simulink model "c_coder"  (R2021b)
settings: Solver=FixedStepAuto  StartTime=0.0  StopTime=inf  FixedStep=0.02  RelTol=1e-3
InitFcn:
  | run('./init_simulink.m');
values from neighbouring files (symbols this model uses):
  qsi = 1    [init_simulink.m]
  w0_acc = 2*pi*f0_acc    (= 0.628318530718)    [init_simulink.m]
  w0_lp = 2*pi*f0_lp    (= 6.28318530718)    [init_simulink.m]
  w0_pos = 2*pi*f0_pos    (= 6.28318530718)    [init_simulink.m]
  w0_vel = 2*pi*f0_vel    (= 1.88495559215)    [init_simulink.m]
undefined symbols (not defined in the file or in its folder): CR, DiscIntNeverNeededParam, LF
libraries: dspstat3 x6, simulink x3, slrealtimeiplib x3, instrumentlib x2, instrumentseriallib x2, etargetslib x1, simulink_extras x1, aerolibanimutils x1, dspnetwork x1
settings Model: Creator=sergi  LastModifiedBy=filip
settings SolverCC: AllowMultiTaskInputOutput=on  AlgebraicLoopSolver=TrustRegion  PositivePriorityOrder=on  AutoInsertRateTranBlk=on
settings DataIOCC: ReturnWorkspaceOutputs=off
settings OptimizationCC: BlockReduction=off  DefaultParameterBehavior=Inlined  EnhancedBackFolding=on  PassReuseOutputArgsAs=Individual arguments  ZeroExternalMemoryAtStartup=off  OptimizeBlockOrder=speed  DifferentSizesBufferReuse=on  OptimizationCustomize=off  EfficientTunableParamExpr=on
settings DebuggingCC: TasksWithSamePriorityMsg=none  ParameterTunabilityLossMsg=error  SFMachineParentedDataDiag=warning  ArithmeticOperatorsInVariantConditions=warning
settings HardwareCC: TargetBitPerPointer=64  TargetBitPerSizeT=64  TargetBitPerPtrDiffT=64  TargetLongLongMode=on  TargetIntDivRoundTo=Zero  TargetEndianess=LittleEndian  TargetWordSize=64  TargetHWDeviceType=MATLAB Host  ProdEqTarget=off
settings SFSimCC: SimUseLocalCustomCode=off  MATLABDynamicMemAlloc=off  CustomCodeUndefinedFunction=UseInterfaceOnly
settings RTWCC: Description=Embedded Coder (host-based shared library target)  SystemTargetFile=ert_shrlib.tlc  TemplateMakefile=ert_default_tmf  GenerateReport=on  RTWUseLocalCustomCode=off  Toolchain=MinGW64 | gmake (64-bit Windows)  BuildConfiguration=Faster Runs  LaunchReport=on  CodeExecutionProfiling=on
settings CodeAppCC: ForceParamTrailComments=on  IgnoreCustomStorageClasses=off  MaxIdLength=95  OperatorAnnotations=on  SimulinkDataObjDesc=on  SFDataObjDesc=on  InsertBlockDesc=on
settings STFCustomTargetCC: TargetLangStandard=C99 (ISO)  MultiwordLength=256  GenerateSampleERTMain=on  ParMdlRefBuildCompliant=on  CompOptLevelCompliant=on  CombineOutputUpdateFcns=on  ERTCustomFileBanners=on  CodeInterfacePackaging=Reusable function  SupportNonInlinedSFcns=off  RemoveResetFunc=on  MATLABClassNameForMDSCustomization=Simulink.SoftwareTarget.ERTCustomization  ModelStepFunctionPrototypeControlCompliant=on  GRTInterface=off  UseToolchainInfoCompliant=on  SystemTargetFile=ert_shrlib.tlc
settings ERTTargetCC: TargetLangStandard=C99 (ISO)  GenerateSampleERTMain=on  ConcurrentExecutionCompliant=off  CodeInterfacePackaging=Reusable function  SupportContinuousTime=on  CPPClassGenCompliant=off  InlinedParameterPlacement=NonHierarchical  ERTCustomFileTemplate=example_file_process.tlc

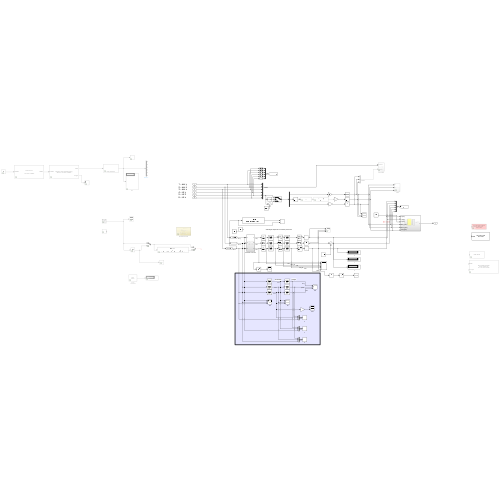
[thumbnail: Simulink's stored preview of the top-level diagram]
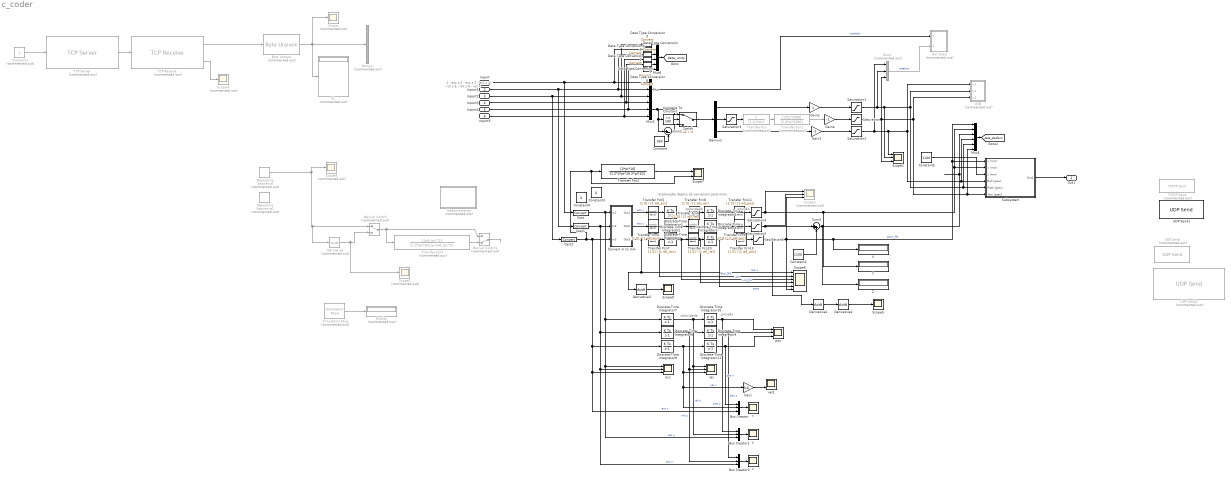
== system c_coder ==
  note: 1 - acc y
      | 2 - acc z
      | 3 - acc x
      | 4 - rot y
      | 5 - rot z
      | 6 - rot x
  note: aceleração depois da conversao para mms
  note: posição
  note: velocidade
  note: posição
  note: velocidade
  Inport : Inport  OutDataTypeStr=double
  Inport1 : Inport  Port=2  OutDataTypeStr=double
  Inport2 : Inport  Port=3  OutDataTypeStr=double
  Inport3 : Inport  Port=4  OutDataTypeStr=double
  Inport4 : Inport  Port=5  OutDataTypeStr=double
  Inport5 : Inport  Port=6  OutDataTypeStr=double
  Bus Creator : BusCreator  Inputs=3
  Bus Creator1 : BusCreator  Inputs=3
  Bus Creator2 : BusCreator  Inputs=3
  Byte Unpack : etargetslib/Byte Unpack  Commented=on  dimensions={[6]}  datatypes={'single'}  byteAlign=1
  Cast : DataTypeConversion
  Cast1 : DataTypeConversion
  Cast2 : DataTypeConversion
  Compare To Constant : simulink/Logic and Bit Operations/Compare To Constant  relop=<=  const=180  OutDataTypeStr=boolean
  Constant : Constant  Value=360
  Constant1 : Constant  Commented=on
  Constant2 : Constant  Value=1100
  Constant3 : Constant  Value=0
  Constant4 : Constant  Value=0
  Constant5 : Constant  Value=1100
  Convert m to mm : Subsystem
  Data Type Conversion{3..8} (6 alike) : DataTypeConversion
  Demux : Demux  Commented=on  Outputs=6
  Demux1 : Demux  Outputs=3
  Derivative : Derivative  Commented=on
  Derivative1 : Derivative
  Derivative2 : Derivative
  Derivative3 : Derivative
  Discrete-Time Integrator{,2..11} (11 alike) : DiscreteIntegrator  SampleTime=-1  UpperSaturationLimit=150  LowerSaturationLimit=-150  ICPrevOutput=DiscIntNeverNeededParam  ICPrevScaledInput=DiscIntNeverNeededParam
  Discrete-Time Integrator1 : DiscreteIntegrator  SampleTime=-1  UpperSaturationLimit=1000  LowerSaturationLimit=-1000  ICPrevOutput=DiscIntNeverNeededParam  ICPrevScaledInput=DiscIntNeverNeededParam
  Display : Display  Commented=on
  Gain : Gain  Gain=3.6
  Gain2 : Gain
  Gain3 : Gain  Gain=-1
  Gain4 : Gain  Gain=-1
  Manual Switch : ManualSwitch  Commented=on
  Manual Switch1 : ManualSwitch  Commented=on  CurrentSetting=0
  Measurements : Subsystem  Commented=on
  Mux : Mux  Inputs=3
  Mux1 : Mux  Commented=on  Inputs=3
  Mux2 : Mux  Inputs=3
  Mux5 : Mux  Inputs=6
  Mux6 : Mux  Inputs=6
  Not Used : Subsystem  Commented=on
  Repeating Sequence : simulink/Sources/Repeating Sequence  Commented=on  rep_seq_t=[0 2 10 17 21 23 30 39 45 50]  rep_seq_y=[0 0 2.4 2.4 -0.33 -0.33 -5.8 -5.8 0 0]
  Repeating Sequence1 : simulink/Sources/Repeating Sequence  Commented=on  rep_seq_t=t_acc  rep_seq_y=v_acc
  Saturation{,1..3} (4 alike) : Saturate  UpperLimit=15  LowerLimit=-15
  Saturation4 : Saturate  UpperLimit=250  LowerLimit=-250
  Saturation5 : Saturate  UpperLimit=250  LowerLimit=-250
  Saturation6 : Saturate  UpperLimit=250  LowerLimit=-250
  Scope{,2,4,8} (4 alike) : Scope  Commented=on
  Scope1 : Scope  NumInputPorts=3
  Scope3 : Scope  Commented=on  NumInputPorts=3
  Scope5 : Scope
  Scope6 : Scope  NumInputPorts=6
  Scope7 : Scope  NumInputPorts=2
  Scope9 : Scope
  Simulation Pace : aerolibanimutils/Simulation Pace  Commented=on  SimulationPace=1  SleepMode=Auto  OutputPaceError=on  SampleTime=0.02
  Subsystem : Subsystem
  Sum2 : Sum  Inputs=|+-
  Sum3 : Sum  Inputs=|++
  Switch : Switch  Criteria=u2 > Threshold
  TCP Receive : slrealtimeiplib/TCP Receive  Commented=on  socketAddPortVal=<empty>  rcvWidth=6*4  sampleTime=-1
      settings: SourceProductBaseCode=XP
  TCP Server : slrealtimeiplib/TCP Server  Priority=-1  Commented=on  useHostTargetConn=off  serverAddress=127.0.0.1  serverPort=55001
      settings: SourceProductBaseCode=XP
  TCP/IP Send : instrumentlib/TCP//IP Send  Commented=on  Host=192.168.0.101  Port=502  ByteOrder=little-endian  EnableBlockingMode=off  Timeout=10  TransferDelay=on  SimulateUsing=Interpreted execution
  Transfer Fcn : TransferFcn  Commented=on  Numerator=[1 0]  Denominator=[1 0.2*pi]
  Transfer Fcn1 : TransferFcn  Commented=on  Numerator=[2*pi*1000]  Denominator=[1 2*pi*1000]
  Transfer Fcn10 : TransferFcn  Numerator=[1 0]  Denominator=[1 w0_vel]
  Transfer Fcn11 : TransferFcn  Numerator=[1 0]  Denominator=[1 w0_pos]
  Transfer Fcn13 : TransferFcn  Numerator=[1 0]  Denominator=[1 w0_pos]
  Transfer Fcn2 : TransferFcn  Numerator=[2*pi*10]  Denominator=[1 2*2*pi*10 2*pi*10]
  Transfer Fcn3 : TransferFcn  Commented=on  Numerator=[(w0_lp)^2]  Denominator=[1 2*qsi*w0_lp (w0_lp)^2]
  Transfer Fcn4 : TransferFcn  Numerator=[1 0]  Denominator=[1 w0_acc]
  Transfer Fcn5 : TransferFcn  Numerator=[1 0]  Denominator=[1 w0_acc]
  Transfer Fcn6 : TransferFcn  Numerator=[1 0]  Denominator=[1 w0_vel]
  Transfer Fcn7 : TransferFcn  Numerator=[1 0]  Denominator=[1 w0_acc]
  Transfer Fcn8 : TransferFcn  Numerator=[1 0]  Denominator=[1 w0_vel]
  Transfer Fcn9 : TransferFcn  Numerator=[1 0]  Denominator=[1 w0_pos]
  UDP Send : dspnetwork/UDP Send  Commented=on  remoteURL='127.0.0.1'  remotePort=25000  localURL='0.0.0.0'  localPortSource=Automatically determine  localPort=-1  sendBufferSize=8192  sampletime=-1  blockPlatform=[]  separateLengthPort=0
  UDP Send1 : instrumentlib/UDP Send  Host=192.168.0.100  Port=502  LocalPort=-1  EnablePortSharing=off  ByteOrder=LittleEndian  OutputDatagramPacketSize=256  EnableBlockingMode=on  LocalAddress=0.0.0.0
  UDP Send2 : slrealtimeiplib/UDP Send  Commented=on  useHostTargetConn=off  toAddress='10.10.10.10'  toPort=34  sampleTime=-1
      settings: SourceProductBaseCode=XP
  USB : Subsystem  Commented=on
  X : Display
  X1 : Display  Commented=on
  Y : Display
  Z : Display
  acc : Scope  NumInputPorts=3
  pos : Scope  NumInputPorts=3
  vel : Scope  NumInputPorts=3
  vel1 : Scope  NumInputPorts=3
  x : Scope
  y : Scope
  z : Scope
  Out1 : Outport
  tag scope: data_platform=global, data_unity=global
  wires:
  Inport5/1 -> Mux2/3, Data Type Conversion6/1
  Inport3/1 -> Data Type Conversion7/1, Mux2/1
  Inport2/1 -> Cast2/1, Mux/3, Data Type Conversion3/1
  Inport1/1 -> Cast1/1, Data Type Conversion5/1, Mux/2
  Inport/1 -> Data Type Conversion4/1, Mux/1, Cast/1
  Mux2/1 -> Switch/1, Sum2/1, Compare To Constant/1
  Constant/1 -> Sum2/2
  Compare To Constant/1 -> Switch/2
  Sum2/1 -> Switch/3
  Demux1/1 -> Gain2/1
  Demux1/3 -> Gain3/1
  Transfer Fcn/1 -> Transfer Fcn1/1
  Demux1/2 -> Saturation3/1
  Saturation1/1 -> Scope1/2, Subsystem/5(Pitch (grau)), Mux5/5, USB/2(In2), Mux1/2
  Saturation2/1 -> Mux1/1, USB/1(In1), Subsystem/4("Roll (grau) "), Mux5/4, Scope1/1
  Gain2/1 -> Saturation1/1
  Gain3/1 -> Saturation2/1
  Saturation3/1 -> Transfer Fcn/1
  Switch/1 -> Demux1/1
  Saturation/1 -> Scope1/3, Subsystem/6(Yaw (grau)), Mux5/6, USB/3(In3), Mux1/3
  Transfer Fcn1/1 -> Gain4/1
  Gain4/1 -> Saturation/1
  Mux5/1 -> [data_platform]
  Inport4/1 -> Data Type Conversion8/1, Mux2/2
  Data Type Conversion3/1 -> Mux6/1
  Data Type Conversion4/1 -> Mux6/2
  Data Type Conversion5/1 -> Mux6/3
  Data Type Conversion6/1 -> Mux6/4
  Data Type Conversion7/1 -> Mux6/5
  Data Type Conversion8/1 -> Mux6/6
  Mux6/1 -> [data_unity]
  Mux/1 -> Not Used/1(position)  "position"
  Mux1/1 -> Not Used/2(rotation)  "rotation"
  Subsystem/1(Out1) -> Out1/1
  Discrete-Time Integrator1/1 -> Transfer Fcn8/1
  Discrete-Time Integrator/1 -> Transfer Fcn6/1
  Discrete-Time Integrator2/1 -> Scope6/3, Transfer Fcn10/1  "velx"
  Discrete-Time Integrator4/1 -> Transfer Fcn11/1
  Discrete-Time Integrator3/1 -> Transfer Fcn9/1
  Discrete-Time Integrator5/1 -> Scope6/5, Transfer Fcn13/1  "posx"
  Cast/1 -> acc/1, Bus Creator1/3, Discrete-Time Integrator7/1, Convert m to mm/1(In1)  "acc y"
  Cast1/1 -> Convert m to mm/2(In2), Bus Creator2/3, acc/2, Discrete-Time Integrator6/1  "acc z"
  Cast2/1 -> Scope7/2, Transfer Fcn2/1, Discrete-Time Integrator8/1, Bus Creator/3, acc/3, Convert m to mm/3(In3)  "acc x"
  Saturation4/1 -> Scope3/1, Y/1, Subsystem/2(y (mm)), Mux5/2
  Sum3/1 -> Mux5/3, Z/1
  Saturation6/1 -> Derivative1/1, Scope3/3, Scope6/6, X/1, Subsystem/1(x (mm)), Mux5/1  "posx_filt"
  Constant2/1 -> Sum3/2
  Saturation5/1 -> Scope3/2, Sum3/1
  Convert m to mm/1(Out1) -> Transfer Fcn5/1  "acc y"
  Convert m to mm/2(Out2) -> Transfer Fcn4/1  "acc z"
  Convert m to mm/3(Out3) -> Scope6/1, Derivative3/1, Transfer Fcn7/1  "acc x"
  TCP Receive/2 -> Scope4/1
  Constant1/1 -> TCP Server/1
  TCP Server/1 -> TCP Receive/1
  Byte Unpack/1 -> Demux/1, Scope/1, X1/1
  Discrete-Time Integrator11/1 -> Bus Creator/1, pos/3  "pos x"
  Discrete-Time Integrator9/1 -> Bus Creator2/1, pos/2  "pos z"
  Discrete-Time Integrator10/1 -> Bus Creator1/1, pos/1  "pos y"
  Discrete-Time Integrator8/1 -> Discrete-Time Integrator11/1, Bus Creator/2, Gain/1, vel/3  "vel x"
  Discrete-Time Integrator6/1 -> Discrete-Time Integrator9/1, Bus Creator2/2, vel/2  "vel z"
  Discrete-Time Integrator7/1 -> Discrete-Time Integrator10/1, Bus Creator1/2, vel/1  "vel y"
  Bus Creator/1 -> x/1
  Bus Creator1/1 -> y/1
  Bus Creator2/1 -> z/1
  Transfer Fcn5/1 -> Discrete-Time Integrator1/1
  Transfer Fcn4/1 -> Discrete-Time Integrator/1
  Transfer Fcn7/1 -> Scope6/2, Discrete-Time Integrator2/1  "accx_filt"
  Transfer Fcn6/1 -> Discrete-Time Integrator3/1
  Transfer Fcn10/1 -> Scope6/4, Discrete-Time Integrator5/1  "vrlx_filt"
  Transfer Fcn8/1 -> Discrete-Time Integrator4/1
  Transfer Fcn13/1 -> Saturation6/1
  Transfer Fcn9/1 -> Saturation5/1
  Transfer Fcn11/1 -> Saturation4/1
  Constant5/1 -> Subsystem/3(z (mm))
  Transfer Fcn2/1 -> Scope7/1
  Repeating Sequence/1 -> Scope8/1, Derivative/1, Manual Switch/1
  Manual Switch/1 -> Manual Switch1/1, Transfer Fcn3/1
  Derivative/1 -> Scope2/1, Manual Switch/2
  Manual Switch1/1 -> ?
  Transfer Fcn3/1 -> Manual Switch1/2
  Derivative1/1 -> Derivative2/1
  Derivative2/1 -> Scope5/1
  Derivative3/1 -> Scope9/1
  Simulation Pace/1 -> Display/1
  Gain/1 -> vel1/3
  TCP Receive/1 -> Byte Unpack/1

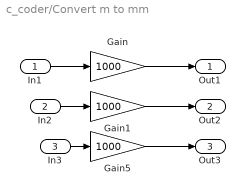
== system c_coder/Convert m to mm ==
  In1 : Inport
  In2 : Inport  Port=2
  In3 : Inport  Port=3
  Gain : Gain  Gain=1000
  Gain1 : Gain  Gain=1000
  Gain5 : Gain  Gain=1000
  Out1 : Outport
  Out2 : Outport  Port=2
  Out3 : Outport  Port=3
  wires:
  Gain/1 -> Out1/1
  Gain5/1 -> Out3/1
  In3/1 -> Gain5/1
  In1/1 -> Gain/1
  In2/1 -> Gain1/1
  Gain1/1 -> Out2/1

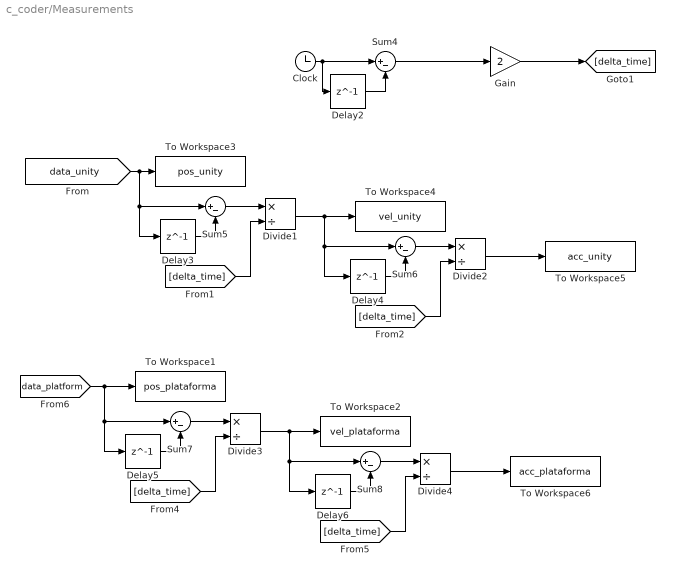
== system c_coder/Measurements ==
  Clock : Clock
  Delay{2..6} (5 alike) : Delay  DelayLength=1
  Divide{1..4} (4 alike) : Product  Inputs=*/
  Gain : Gain  Gain=2
  Sum{4..8} (5 alike) : Sum  Inputs=|+-
  To Workspace1 : ToWorkspace  VariableName=pos_plataforma  SaveFormat=Structure With Time  SampleTime=-1
  To Workspace2 : ToWorkspace  VariableName=vel_plataforma  SaveFormat=Structure With Time  SampleTime=-1
  To Workspace3 : ToWorkspace  VariableName=pos_unity  SaveFormat=Structure With Time  SampleTime=-1
  To Workspace4 : ToWorkspace  VariableName=vel_unity  SaveFormat=Structure With Time  SampleTime=-1
  To Workspace5 : ToWorkspace  VariableName=acc_unity  SaveFormat=Structure With Time  SampleTime=-1
  To Workspace6 : ToWorkspace  VariableName=acc_plataforma  SaveFormat=Structure With Time  SampleTime=-1
  wires:
  Divide3/1 -> To Workspace2/1, Delay6/1, Sum8/1
  Divide2/1 -> To Workspace5/1
  Sum5/1 -> Divide1/1
  [delta_time] -> Divide1/2
  [data_unity] -> Delay3/1, Sum5/1, To Workspace3/1
  Delay2/1 -> Sum4/2
  Clock/1 -> Delay2/1, Sum4/1
  Delay3/1 -> Sum5/2
  [delta_time] -> Divide3/2
  [data_platform] -> To Workspace1/1, Sum7/1, Delay5/1
  Delay4/1 -> Sum6/2
  Divide1/1 -> Sum6/1, Delay4/1, To Workspace4/1
  Sum6/1 -> Divide2/1
  Sum7/1 -> Divide3/1
  [delta_time] -> Divide2/2
  Sum4/1 -> Gain/1
  [delta_time] -> Divide4/2
  Delay6/1 -> Sum8/2
  Divide4/1 -> To Workspace6/1
  Sum8/1 -> Divide4/1
  Delay5/1 -> Sum7/2
  Gain/1 -> [delta_time]

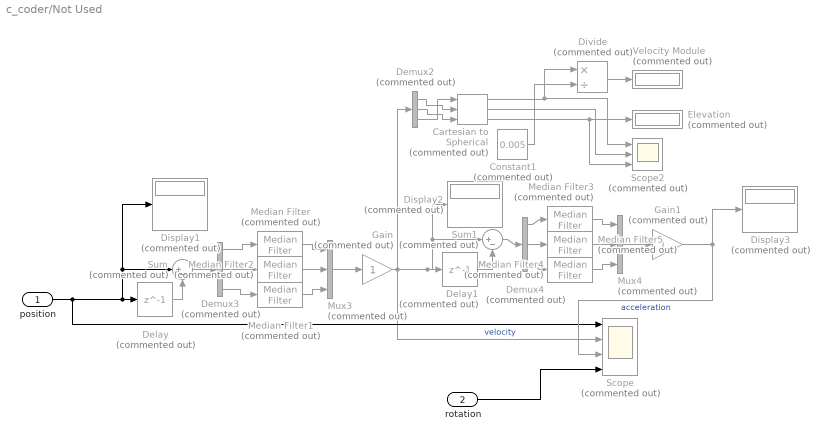
== system c_coder/Not Used ==
  position : Inport
  rotation : Inport  Port=2
  Cartesian to Spherical : simulink_extras/Transformations/Cartesian to Spherical  Commented=on
      settings: SourceProductBaseCode=SL
  Constant1 : Constant  Commented=on  Value=0.005
  Delay : Delay  Commented=on  DelayLength=1
  Delay1 : Delay  Commented=on  DelayLength=1
  Demux2 : Demux  Commented=on  Outputs=3
  Demux3 : Demux  Commented=on  Outputs=3
  Demux4 : Demux  Commented=on  Outputs=3
  Display1 : Display  Commented=on
  Display2 : Display  Commented=on
  Display3 : Display  Commented=on
  Divide : Product  Commented=on  Inputs=*/
  Elevation : Display  Commented=on
  Gain : Gain  Commented=on
  Gain1 : Gain  Commented=on
  Median Filter{,1..5} (6 alike) : dspstat3/Median Filter  Commented=on  WindowLength=10  SimulateUsing=Interpreted execution
      settings: SourceProductName=DSP System Toolbox
  Mux3 : Mux  Commented=on  Inputs=3
  Mux4 : Mux  Commented=on  Inputs=3
  Scope : Scope  Commented=on  NumInputPorts=4
  Scope2 : Scope  Commented=on  NumInputPorts=3
  Sum : Sum  Commented=on  Inputs=|+-
  Sum1 : Sum  Commented=on  Inputs=|+-
  Velocity Module : Display  Commented=on
  wires:
  Gain/1 -> Demux2/1, Scope/2, Display2/1, Sum1/1, Delay1/1  "velocity"
  Cartesian to Spherical/3 -> Scope2/3, Elevation/1
  position/1 -> Scope/1, Delay/1, Display1/1, Sum/1
  Delay/1 -> Sum/2
  Demux2/2 -> Cartesian to Spherical/3
  Demux3/3 -> Median Filter1/1
  Median Filter1/1 -> Mux3/3
  Median Filter4/1 -> Mux4/3
  Cartesian to Spherical/1 -> Scope2/1, Divide/1
  Gain1/1 -> Display3/1, Scope/3  "acceleration"
  Delay1/1 -> Sum1/2
  Demux3/2 -> Median Filter2/1
  Demux2/1 -> Cartesian to Spherical/2
  Demux3/1 -> Median Filter/1
  Sum/1 -> Demux3/1
  Median Filter5/1 -> Mux4/2
  Demux4/3 -> Median Filter4/1
  Mux3/1 -> Gain/1
  Mux4/1 -> Gain1/1
  Constant1/1 -> Divide/2
  Median Filter2/1 -> Mux3/2
  Demux2/3 -> Cartesian to Spherical/1
  Demux4/2 -> Median Filter5/1
  Sum1/1 -> Demux4/1
  Median Filter3/1 -> Mux4/1
  Median Filter/1 -> Mux3/1
  Demux4/1 -> Median Filter3/1
  Divide/1 -> Velocity Module/1
  Cartesian to Spherical/2 -> Scope2/2
  rotation/1 -> Scope/4

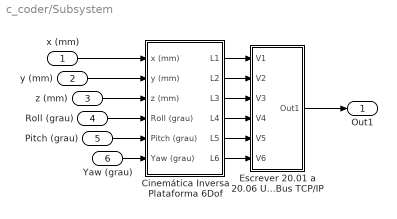
== system c_coder/Subsystem ==
  x (mm) : Inport
  y (mm) : Inport  Port=2
  z (mm) : Inport  Port=3
  "Roll (grau) " : Inport  Port=4
  Pitch (grau) : Inport  Port=5
  Yaw (grau) : Inport  Port=6
  Cinemática Inversa Plataforma 6Dof : Subsystem  mask(Cinemática Inversa - Plataforma 6DOF){a=180, b=180, c=1200, d=210, e=220, f=690, Lmin=750, Gs=10}
      mask prompts: a "Constante 'a' (mm)"; b "Constante 'b' (mm)"; c "Constante 'c' (mm)"; d "Constante 'd' (mm)"; e "Constante 'e (mm)"; f "Constante 'f' (mm)"; Lmin "Constante 'Lmin' (mm)"; Gs "Ganho de saida 'Gs'"
      mask help: Modelo da cinemática inversa de uma plataforma de Gough-Stewart do tipo 6-6
  Escrever 20.01 a 20.06 UNIDRIVE SP ModBus TCP/IP : Subsystem
  Out1 : Outport
  wires:
  Yaw (grau)/1 -> Cinemática Inversa Plataforma 6Dof/6(Yaw (grau))
  Cinemática Inversa Plataforma 6Dof/1(L1) -> Escrever 20.01 a 20.06 UNIDRIVE SP ModBus TCP/IP/1(V1)
  Escrever 20.01 a 20.06 UNIDRIVE SP ModBus TCP/IP/1(Out1) -> Out1/1
  Cinemática Inversa Plataforma 6Dof/2(L2) -> Escrever 20.01 a 20.06 UNIDRIVE SP ModBus TCP/IP/2(V2)
  Pitch (grau)/1 -> Cinemática Inversa Plataforma 6Dof/5(Pitch (grau))
  Cinemática Inversa Plataforma 6Dof/6(L6) -> Escrever 20.01 a 20.06 UNIDRIVE SP ModBus TCP/IP/6(V6)
  Cinemática Inversa Plataforma 6Dof/4(L4) -> Escrever 20.01 a 20.06 UNIDRIVE SP ModBus TCP/IP/4(V4)
  Cinemática Inversa Plataforma 6Dof/3(L3) -> Escrever 20.01 a 20.06 UNIDRIVE SP ModBus TCP/IP/3(V3)
  Cinemática Inversa Plataforma 6Dof/5(L5) -> Escrever 20.01 a 20.06 UNIDRIVE SP ModBus TCP/IP/5(V5)
  z (mm)/1 -> Cinemática Inversa Plataforma 6Dof/3(z (mm))
  "Roll (grau) "/1 -> Cinemática Inversa Plataforma 6Dof/4("Roll (grau) ")
  x (mm)/1 -> Cinemática Inversa Plataforma 6Dof/1(x (mm))
  y (mm)/1 -> Cinemática Inversa Plataforma 6Dof/2(y (mm))

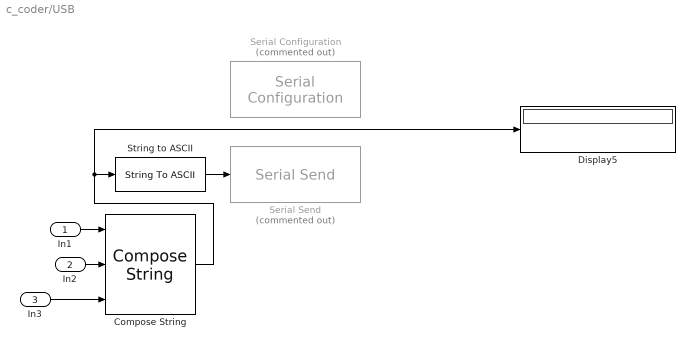
== system c_coder/USB ==
  In1 : Inport
  In2 : Inport  Port=2
  In3 : Inport  Port=3
  Compose String : ComposeString  Format="\"P;0;0;0;%0.1f;%0.1f;%0.1f\""
  Display5 : Display
  Serial Configuration : instrumentseriallib/Serial Configuration  Priority=-200000  Commented=on  Port=<Select a port...>  ComPort=<Select a port...>  BaudRate=19200  DataBits=8  Parity=none  StopBits=1  ByteOrder=little-endian  FlowControl=none  Timeout=1  SimulateUsing=Interpreted execution  BlockInModel=on
  Serial Send : instrumentseriallib/Serial Send  Commented=on  Port=<Select a port...>  ComPort=COM22  Header=[]  Terminator=CR/LF ('\r\n')  CustomTerminator=[]  EnableBlockingMode=off  SimulateUsing=Interpreted execution  BlockInModel=on
  String to ASCII : StringToASCII
  wires:
  Compose String/1 -> String to ASCII/1, Display5/1
  String to ASCII/1 -> Serial Send/1
  In1/1 -> Compose String/1
  In2/1 -> Compose String/2
  In3/1 -> Compose String/3

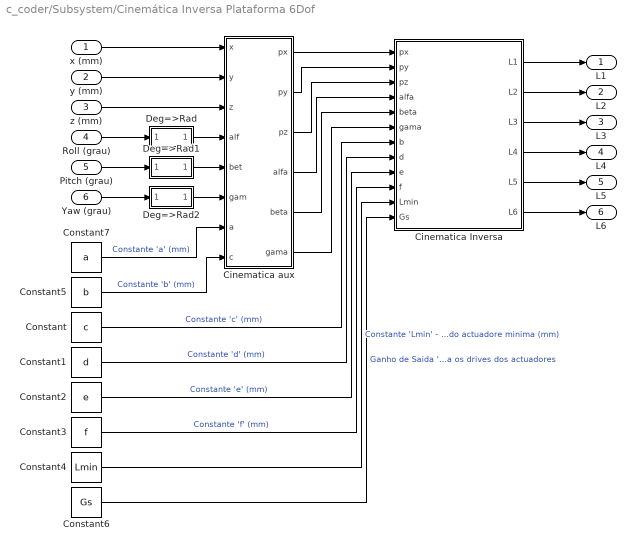
== system c_coder/Subsystem/Cinemática Inversa Plataforma 6Dof ==
  x (mm) : Inport
  y (mm) : Inport  Port=2
  z (mm) : Inport  Port=3
  "Roll (grau) " : Inport  Port=4
  Pitch (grau) : Inport  Port=5
  Yaw (grau) : Inport  Port=6
  Cinematica aux : Subsystem
  Cinematica Inversa : Subsystem
  Constant : Constant  Value=c
  Constant1 : Constant  Value=d
  Constant2 : Constant  Value=e
  Constant3 : Constant  Value=f
  Constant4 : Constant  Value=Lmin
  Constant5 : Constant  Value=b
  Constant6 : Constant  Value=Gs
  Constant7 : Constant  Value=a
  Deg=>Rad : Subsystem
  Deg=>Rad1 : Subsystem
  Deg=>Rad2 : Subsystem
  L1 : Outport  SampleTime=0.02
  L2 : Outport  Port=2  SampleTime=0.02
  L3 : Outport  Port=3  SampleTime=0.02
  L4 : Outport  Port=4  SampleTime=0.02
  L5 : Outport  Port=5  SampleTime=0.02
  L6 : Outport  Port=6  SampleTime=0.02
  wires:
  Deg=>Rad/1(Rad) -> Cinematica aux/4(alf)
  Constant/1 -> Cinematica Inversa/7(b)  "Constante 'c' (mm)"
  Constant1/1 -> Cinematica Inversa/8(d)  "Constante 'd' (mm)"
  Constant2/1 -> Cinematica Inversa/9(e)  "Constante 'e' (mm)"
  Constant3/1 -> Cinematica Inversa/10(f)  "Constante 'f' (mm)"
  Constant4/1 -> Cinematica Inversa/11(Lmin)  "Constante 'Lmin' - Comprimento do actuadore minima (mm)"
  Cinematica aux/4(alfa) -> Cinematica Inversa/4(alfa)
  Deg=>Rad1/1(Rad) -> Cinematica aux/5(bet)
  Deg=>Rad2/1(Rad) -> Cinematica aux/6(gam)
  Constant6/1 -> Cinematica Inversa/12(Gs)  "Ganho de Saida 'Gs' - Ganho de saida para os drives dos actuadores"
  Constant7/1 -> Cinematica aux/7(a)  "Constante 'a' (mm)"
  Constant5/1 -> Cinematica aux/8(c)  "Constante 'b' (mm)"
  Cinematica aux/6(gama) -> Cinematica Inversa/6(gama)
  Cinematica aux/5(beta) -> Cinematica Inversa/5(beta)
  Cinematica aux/3(pz) -> Cinematica Inversa/3(pz)
  Cinematica aux/2(py) -> Cinematica Inversa/2(py)
  Cinematica aux/1(px) -> Cinematica Inversa/1(px)
  x (mm)/1 -> Cinematica aux/1(x)
  Cinematica Inversa/1(L1) -> L1/1
  y (mm)/1 -> Cinematica aux/2(y)
  Cinematica Inversa/2(L2) -> L2/1
  z (mm)/1 -> Cinematica aux/3(z)
  Cinematica Inversa/3(L3) -> L3/1
  "Roll (grau) "/1 -> Deg=>Rad/1(Deg)
  Cinematica Inversa/4(L4) -> L4/1
  Pitch (grau)/1 -> Deg=>Rad1/1(Deg)
  Cinematica Inversa/5(L5) -> L5/1
  Yaw (grau)/1 -> Deg=>Rad2/1(Deg)
  Cinematica Inversa/6(L6) -> L6/1

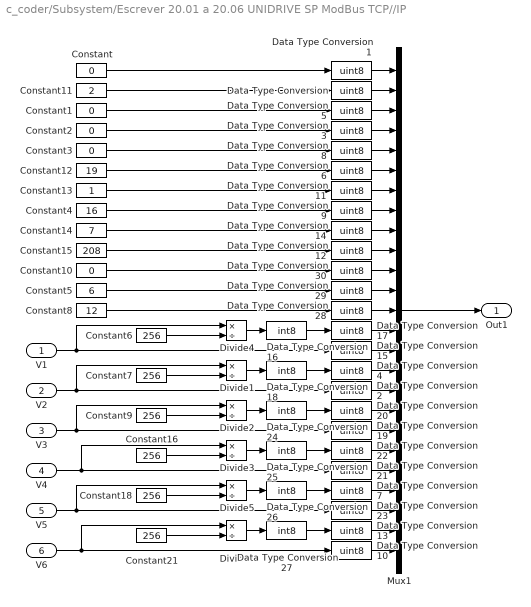
== system c_coder/Subsystem/Escrever 20.01 a 20.06 UNIDRIVE SP ModBus TCP//IP ==
  V1 : Inport
  V2 : Inport  Port=2
  V3 : Inport  Port=3
  V4 : Inport  Port=4
  V5 : Inport  Port=5
  V6 : Inport  Port=6
  Constant{,1..3,10} (5 alike) : Constant  Value=0
  Constant11 : Constant  Value=2
  Constant12 : Constant  Value=19
  Constant13 : Constant
  Constant14 : Constant  Value=7
  Constant15 : Constant  Value=208
  Constant{6..7,9,16,18,21} (6 alike) : Constant  Value=256
  Constant4 : Constant  Value=16
  Constant5 : Constant  Value=6
  Constant8 : Constant  Value=12
  Data Type Conversion{,1..15,17,19..23,28..30} (25 alike) : DataTypeConversion  OutDataTypeStr=uint8
  Data Type Conversion{16,18,24..27} (6 alike) : DataTypeConversion  OutDataTypeStr=int8
  Divide{1..6} (6 alike) : Product  Inputs=*/
  Mux1 : Mux  Inputs=25
  Out1 : Outport
  wires:
  Data Type Conversion1/1 -> Mux1/1
  Data Type Conversion/1 -> Mux1/2
  Data Type Conversion5/1 -> Mux1/3
  Data Type Conversion3/1 -> Mux1/4
  Data Type Conversion6/1 -> Mux1/6
  Data Type Conversion11/1 -> Mux1/7
  Data Type Conversion9/1 -> Mux1/8
  Data Type Conversion14/1 -> Mux1/9
  Data Type Conversion12/1 -> Mux1/10
  Data Type Conversion17/1 -> Mux1/14
  Data Type Conversion15/1 -> Mux1/15
  Data Type Conversion8/1 -> Mux1/5
  Constant/1 -> Data Type Conversion1/1
  Constant11/1 -> Data Type Conversion/1
  Constant13/1 -> Data Type Conversion11/1
  Constant14/1 -> Data Type Conversion14/1
  Constant15/1 -> Data Type Conversion12/1
  Data Type Conversion4/1 -> Mux1/16
  Data Type Conversion2/1 -> Mux1/17
  Data Type Conversion20/1 -> Mux1/18
  Data Type Conversion19/1 -> Mux1/19
  Data Type Conversion22/1 -> Mux1/20
  Data Type Conversion21/1 -> Mux1/21
  Data Type Conversion7/1 -> Mux1/22
  Data Type Conversion23/1 -> Mux1/23
  Data Type Conversion13/1 -> Mux1/24
  Data Type Conversion10/1 -> Mux1/25
  Divide4/1 -> Data Type Conversion16/1
  Data Type Conversion16/1 -> Data Type Conversion17/1
  V1/1 -> Divide4/1, Data Type Conversion15/1
  Constant12/1 -> Data Type Conversion6/1
  Constant6/1 -> Divide4/2
  Constant4/1 -> Data Type Conversion9/1
  Constant3/1 -> Data Type Conversion8/1
  Constant2/1 -> Data Type Conversion3/1
  Constant1/1 -> Data Type Conversion5/1
  Divide1/1 -> Data Type Conversion18/1
  Data Type Conversion18/1 -> Data Type Conversion4/1
  V2/1 -> Data Type Conversion2/1, Divide1/1
  Constant7/1 -> Divide1/2
  Divide2/1 -> Data Type Conversion24/1
  Data Type Conversion24/1 -> Data Type Conversion20/1
  V3/1 -> Data Type Conversion19/1, Divide2/1
  Constant9/1 -> Divide2/2
  Divide3/1 -> Data Type Conversion25/1
  Data Type Conversion25/1 -> Data Type Conversion22/1
  V4/1 -> Data Type Conversion21/1, Divide3/1
  Constant16/1 -> Divide3/2
  Divide5/1 -> Data Type Conversion26/1
  Data Type Conversion26/1 -> Data Type Conversion7/1
  V5/1 -> Data Type Conversion23/1, Divide5/1
  Constant18/1 -> Divide5/2
  Divide6/1 -> Data Type Conversion27/1
  Data Type Conversion27/1 -> Data Type Conversion13/1
  V6/1 -> Data Type Conversion10/1, Divide6/1
  Constant21/1 -> Divide6/2
  Data Type Conversion30/1 -> Mux1/11
  Data Type Conversion29/1 -> Mux1/12
  Data Type Conversion28/1 -> Mux1/13
  Constant5/1 -> Data Type Conversion29/1
  Constant8/1 -> Data Type Conversion28/1
  Constant10/1 -> Data Type Conversion30/1
  Mux1/1 -> Out1/1

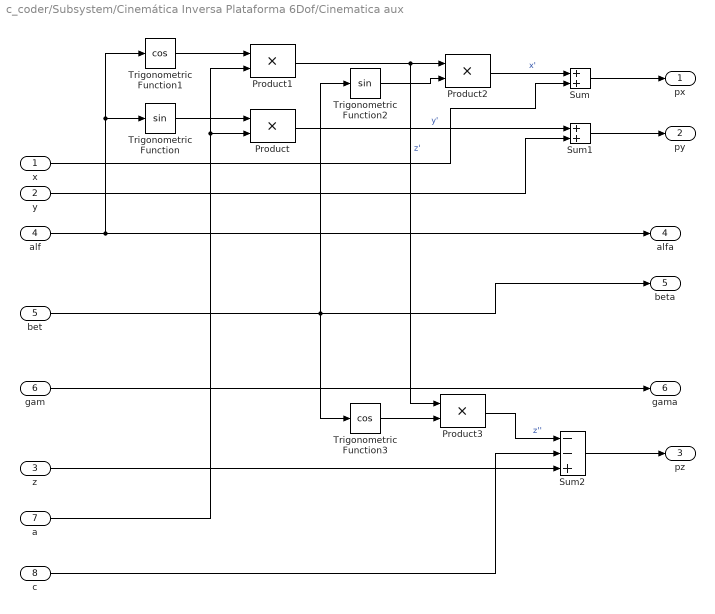
== system c_coder/Subsystem/Cinemática Inversa Plataforma 6Dof/Cinematica aux ==
  x : Inport
  y : Inport  Port=2
  z : Inport  Port=3
  alf : Inport  Port=4
  bet : Inport  Port=5
  gam : Inport  Port=6
  a : Inport  Port=7
  c : Inport  Port=8
  Product{,1..3} (4 alike) : Product  SaturateOnIntegerOverflow=on  OutDataTypeStr=Inherit: Same as first input
  Sum : Sum  SaturateOnIntegerOverflow=on
  Sum1 : Sum  SaturateOnIntegerOverflow=on
  Sum2 : Sum  Inputs=--+  SaturateOnIntegerOverflow=on
  Trigonometric Function : Trigonometry
  Trigonometric Function1 : Trigonometry  Operator=cos
  Trigonometric Function2 : Trigonometry
  Trigonometric Function3 : Trigonometry  Operator=cos
  px : Outport
  py : Outport  Port=2
  pz : Outport  Port=3
  alfa : Outport  Port=4
  beta : Outport  Port=5
  gama : Outport  Port=6
  wires:
  gam/1 -> gama/1
  bet/1 -> Trigonometric Function2/1, Trigonometric Function3/1, beta/1
  alf/1 -> Trigonometric Function/1, Trigonometric Function1/1, alfa/1
  a/1 -> Product1/2, Product/2
  Trigonometric Function1/1 -> Product1/1
  x/1 -> Sum/2
  Sum1/1 -> py/1
  Product/1 -> Sum1/1  "y'"
  y/1 -> Sum1/2
  Sum/1 -> px/1
  Product1/1 -> Product3/1, Product2/1  "z'"
  Product2/1 -> Sum/1  "x'"
  Trigonometric Function3/1 -> Product3/2
  c/1 -> Sum2/2
  Sum2/1 -> pz/1
  Trigonometric Function/1 -> Product/1
  Trigonometric Function2/1 -> Product2/2
  Product3/1 -> Sum2/1  "z''"
  z/1 -> Sum2/3

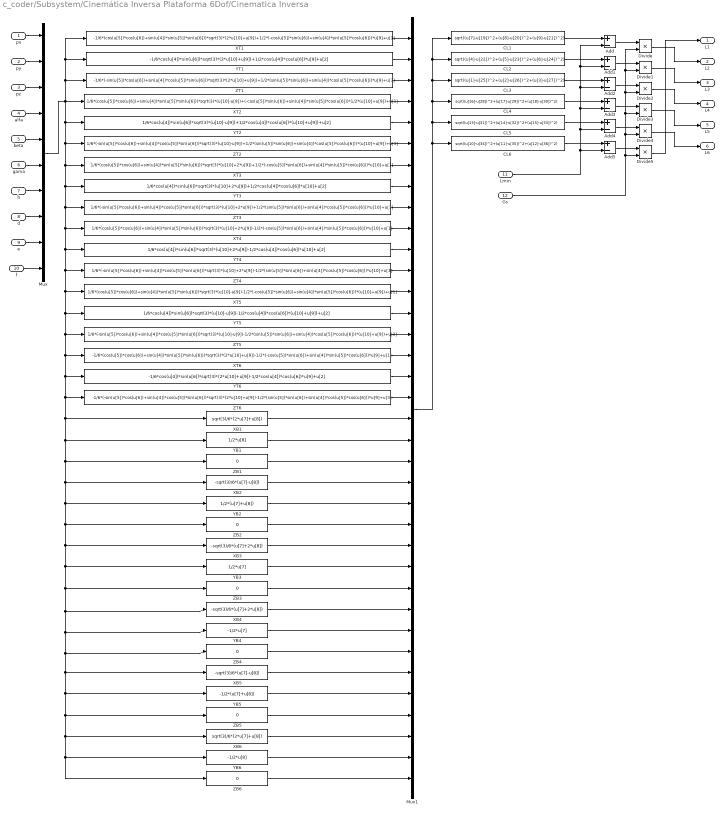
== system c_coder/Subsystem/Cinemática Inversa Plataforma 6Dof/Cinematica Inversa ==
  px : Inport
  py : Inport  Port=2
  pz : Inport  Port=3
  alfa : Inport  Port=4
  beta : Inport  Port=5
  gama : Inport  Port=6
  b : Inport  Port=7
  d : Inport  Port=8
  e : Inport  Port=9
  f : Inport  Port=10
  Lmin : Inport  Port=11
  Gs : Inport  Port=12
  Add{,1..5} (6 alike) : Sum  Inputs=+-
  CL1 : Fcn  Expr=sqrt((u[7]-u[19])^2+(u[8]-u[20])^2+(u[9]-u[21])^2)
  CL2 : Fcn  Expr=sqrt((u[4]-u[22])^2+(u[5]-u[23])^2+(u[6]-u[24])^2)
  CL3 : Fcn  Expr=sqrt((u[1]-u[25])^2+(u[2]-u[26])^2+(u[3]-u[27])^2)
  CL4 : Fcn  Expr=sqrt((u[16]-u[28])^2+(u[17]-u[29])^2+(u[18]-u[30])^2)
  CL5 : Fcn  Expr=sqrt((u[13]-u[31])^2+(u[14]-u[32])^2+(u[15]-u[33])^2)
  CL6 : Fcn  Expr=sqrt((u[10]-u[34])^2+(u[11]-u[35])^2+(u[12]-u[36])^2)
  Divide{,1..5} (6 alike) : Product  Inputs=**
  Mux : Mux  Inputs=10
  Mux1 : Mux  Inputs=36
  XB1 : Fcn  Expr=sqrt(3)/6*(2*u[7]+u[8])
  XB2 : Fcn  Expr=-sqrt(3)/6*(u[7]-u[8])
  XB3 : Fcn  Expr=-sqrt(3)/6*(u[7]+2*u[8])
  XB4 : Fcn  Expr=-sqrt(3)/6*(u[7]+2*u[8])
  XB5 : Fcn  Expr=-sqrt(3)/6*(u[7]-u[8])
  XB6 : Fcn  Expr=sqrt(3)/6*(2*u[7]+u[8])
  XT1 : Fcn  Expr=-1/6*(cos(u[5])*cos(u[6])+sin(u[4])*sin(u[5])*sin(u[6]))*sqrt(3)*(2*u[10]+u[9])+1/2*(-cos(u[5])*sin(u[6])+sin(u[4])*sin(u[5])*cos(u[6]))*u[9]+u[1]
  XT2 : Fcn  Expr=1/6*(cos(u[5])*cos(u[6])+sin(u[4])*sin(u[5])*sin(u[6]))*sqrt(3)*(u[10]-u[9])+(-cos(u[5])*sin(u[6])+sin(u[4])*sin(u[5])*cos(u[6]))*1/2*(u[10]+u[9])+u[1]
  XT3 : Fcn  Expr=1/6*(cos(u[5])*cos(u[6])+sin(u[4])*sin(u[5])*sin(u[6]))*sqrt(3)*(u[10]+2*u[9])+1/2*(-cos(u[5])*sin(u[6])+sin(u[4])*sin(u[5])*cos(u[6]))*u[10]+u[1]
  XT4 : Fcn  Expr=1/6*(cos(u[5])*cos(u[6])+sin(u[4])*sin(u[5])*sin(u[6]))*sqrt(3)*(u[10]+2*u[9])-1/2*(-cos(u[5])*sin(u[6])+sin(u[4])*sin(u[5])*cos(u[6]))*u[10]+u[1]
  XT5 : Fcn  Expr=1/6*(cos(u[5])*cos(u[6])+sin(u[4])*sin(u[5])*sin(u[6]))*sqrt(3)*(u[10]-u[9])-1/2*(-cos(u[5])*sin(u[6])+sin(u[4])*sin(u[5])*cos(u[6]))*(u[10]+u[9])+u[1]
  XT6 : Fcn  Expr=-1/6*(cos(u[5])*cos(u[6])+sin(u[4])*sin(u[5])*sin(u[6]))*sqrt(3)*(2*u[10]+u[9])-1/2*(-cos(u[5])*sin(u[6])+sin(u[4])*sin(u[5])*cos(u[6]))*u[9]+u[1]
  YB1 : Fcn  Expr=1/2*u[8]
  YB2 : Fcn  Expr=1/2*(u[7]+u[8])
  YB3 : Fcn  Expr=1/2*u[7]
  YB4 : Fcn  Expr=-1/2*u[7]
  YB5 : Fcn  Expr=-1/2*(u[7]+u[8])
  YB6 : Fcn  Expr=-1/2*u[8]
  YT1 : Fcn  Expr=-1/6*cos(u[4])*sin(u[6])*sqrt(3)*(2*u[10]+u[9])+1/2*cos(u[4])*cos(u[6])*u[9]+u[2]
  YT2 : Fcn  Expr=1/6*cos(u[4])*sin(u[6])*sqrt(3)*(u[10]-u[9])+1/2*cos(u[4])*cos(u[6])*(u[10]+u[9])+u[2]
  YT3 : Fcn  Expr=1/6*cos(u[4])*sin(u[6])*sqrt(3)*(u[10]+2*u[9])+1/2*cos(u[4])*cos(u[6])*u[10]+u[2]
  YT4 : Fcn  Expr=1/6*cos(u[4])*sin(u[6])*sqrt(3)*(u[10]+2*u[9])-1/2*cos(u[4])*cos(u[6])*u[10]+u[2]
  YT5 : Fcn  Expr=1/6*cos(u[4])*sin(u[6])*sqrt(3)*(u[10]-u[9])-1/2*cos(u[4])*cos(u[6])*(u[10]+u[9])+u[2]
  YT6 : Fcn  Expr=-1/6*cos(u[4])*sin(u[6])*sqrt(3)*(2*u[10]+u[9])-1/2*cos(u[4])*cos(u[6])*u[9]+u[2]
  ZB{1..6} (6 alike) : Fcn  Expr=0
  ZT1 : Fcn  Expr=-1/6*(-sin(u[5])*cos(u[6])+sin(u[4])*cos(u[5])*sin(u[6]))*sqrt(3)*(2*u[10]+u[9])+1/2*(sin(u[5])*sin(u[6])+sin(u[4])*cos(u[5])*cos(u[6]))*u[9]+u[3]
  ZT2 : Fcn  Expr=1/6*(-sin(u[5])*cos(u[6])+sin(u[4])*cos(u[5])*sin(u[6]))*sqrt(3)*(u[10]-u[9])+1/2*(sin(u[5])*sin(u[6])+sin(u[4])*cos(u[5])*cos(u[6]))*(u[10]+u[9])+u[3]
  ZT3 : Fcn  Expr=1/6*(-sin(u[5])*cos(u[6])+sin(u[4])*cos(u[5])*sin(u[6]))*sqrt(3)*(u[10]+2*u[9])+1/2*(sin(u[5])*sin(u[6])+sin(u[4])*cos(u[5])*cos(u[6]))*u[10]+u[3]
  ZT4 : Fcn  Expr=1/6*(-sin(u[5])*cos(u[6])+sin(u[4])*cos(u[5])*sin(u[6]))*sqrt(3)*(u[10]+2*u[9])-1/2*(sin(u[5])*sin(u[6])+sin(u[4])*cos(u[5])*cos(u[6]))*u[10]+u[3]
  ZT5 : Fcn  Expr=1/6*(-sin(u[5])*cos(u[6])+sin(u[4])*cos(u[5])*sin(u[6]))*sqrt(3)*(u[10]-u[9])-1/2*(sin(u[5])*sin(u[6])+sin(u[4])*cos(u[5])*cos(u[6]))*(u[10]+u[9])+u[3]
  ZT6 : Fcn  Expr=-1/6*(-sin(u[5])*cos(u[6])+sin(u[4])*cos(u[5])*sin(u[6]))*sqrt(3)*(2*u[10]+u[9])-1/2*(sin(u[5])*sin(u[6])+sin(u[4])*cos(u[5])*cos(u[6]))*u[9]+u[3]
  L1 : Outport
  L2 : Outport  Port=2
  L3 : Outport  Port=3
  L4 : Outport  Port=4
  L5 : Outport  Port=5
  L6 : Outport  Port=6
  wires:
  px/1 -> Mux/1
  py/1 -> Mux/2
  pz/1 -> Mux/3
  alfa/1 -> Mux/4
  beta/1 -> Mux/5
  gama/1 -> Mux/6
  Mux/1 -> XT2/1, YT2/1, ZT2/1, XT3/1, YT3/1, ZT3/1, XT4/1, YT4/1, ZT4/1, XT5/1, YT5/1, ZT5/1, XT6/1, YT6/1, ZT6/1, XB1/1, YB1/1, ZB1/1, XB2/1, YB2/1, ZB2/1, XB3/1, YB3/1, ZB3/1, XB4/1, YB4/1, ZB4/1, XB5/1, YB5/1, ZB5/1, XB6/1, YB6/1, ZB6/1, XT1/1, YT1/1, ZT1/1
  XT1/1 -> Mux1/1
  YT1/1 -> Mux1/2
  ZT1/1 -> Mux1/3
  XT2/1 -> Mux1/4
  YT2/1 -> Mux1/5
  ZT2/1 -> Mux1/6
  XT3/1 -> Mux1/7
  YT3/1 -> Mux1/8
  ZT3/1 -> Mux1/9
  XT4/1 -> Mux1/10
  YT4/1 -> Mux1/11
  ZT4/1 -> Mux1/12
  XT5/1 -> Mux1/13
  YT5/1 -> Mux1/14
  ZT5/1 -> Mux1/15
  XT6/1 -> Mux1/16
  YT6/1 -> Mux1/17
  ZT6/1 -> Mux1/18
  Mux1/1 -> CL1/1, CL2/1, CL3/1, CL4/1, CL5/1, CL6/1
  b/1 -> Mux/7
  d/1 -> Mux/8
  e/1 -> Mux/9
  f/1 -> Mux/10
  Lmin/1 -> Add5/2, Add4/2, Add3/2, Add2/2, Add1/2, Add/2
  ZB6/1 -> Mux1/36
  XB1/1 -> Mux1/19
  YB1/1 -> Mux1/20
  ZB1/1 -> Mux1/21
  XB2/1 -> Mux1/22
  YB2/1 -> Mux1/23
  ZB2/1 -> Mux1/24
  XB3/1 -> Mux1/25
  YB3/1 -> Mux1/26
  ZB3/1 -> Mux1/27
  XB4/1 -> Mux1/28
  YB4/1 -> Mux1/29
  ZB4/1 -> Mux1/30
  XB5/1 -> Mux1/31
  YB5/1 -> Mux1/32
  ZB5/1 -> Mux1/33
  XB6/1 -> Mux1/34
  YB6/1 -> Mux1/35
  CL1/1 -> Add/1
  CL2/1 -> Add1/1
  CL3/1 -> Add2/1
  CL4/1 -> Add3/1
  CL5/1 -> Add4/1
  CL6/1 -> Add5/1
  Add/1 -> Divide/1
  Divide/1 -> L2/1
  Add1/1 -> Divide1/1
  Divide1/1 -> L3/1
  Add2/1 -> Divide2/1
  Divide2/1 -> L4/1
  Add3/1 -> Divide3/1
  Divide3/1 -> L5/1
  Add4/1 -> Divide4/1
  Divide4/1 -> L6/1
  Add5/1 -> Divide5/1
  Divide5/1 -> L1/1
  Gs/1 -> Divide5/2, Divide4/2, Divide3/2, Divide2/2, Divide1/2, Divide/2

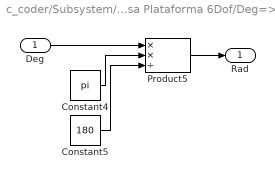
== system c_coder/Subsystem/Cinemática Inversa Plataforma 6Dof/Deg=>Rad ==
  Deg : Inport
  Constant4 : Constant  Value=pi
  Constant5 : Constant  Value=180
  Product5 : Product  Inputs=**/  SaturateOnIntegerOverflow=on  OutDataTypeStr=Inherit: Same as first input
  Rad : Outport
  wires:
  Constant5/1 -> Product5/3
  Constant4/1 -> Product5/2
  Deg/1 -> Product5/1
  Product5/1 -> Rad/1

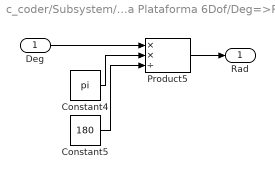
== system c_coder/Subsystem/Cinemática Inversa Plataforma 6Dof/Deg=>Rad1 ==
  Deg : Inport
  Constant4 : Constant  Value=pi
  Constant5 : Constant  Value=180
  Product5 : Product  Inputs=**/  SaturateOnIntegerOverflow=on  OutDataTypeStr=Inherit: Same as first input
  Rad : Outport
  wires:
  Product5/1 -> Rad/1
  Deg/1 -> Product5/1
  Constant4/1 -> Product5/2
  Constant5/1 -> Product5/3

== system c_coder/Subsystem/Cinemática Inversa Plataforma 6Dof/Deg=>Rad2 ==
  Deg : Inport
  Constant4 : Constant  Value=pi
  Constant5 : Constant  Value=180
  Product5 : Product  Inputs=**/  SaturateOnIntegerOverflow=on  OutDataTypeStr=Inherit: Same as first input
  Rad : Outport
  wires:
  Constant5/1 -> Product5/3
  Constant4/1 -> Product5/2
  Deg/1 -> Product5/1
  Product5/1 -> Rad/1
